simulink model "diabetes_2sim"  (R2019a)
settings: Solver=ode45  StartTime=0.0  StopTime=24  RelTol=1e-3  EnableMultiTasking=on
StopFcn:
  | plot_results
libraries: simulink x2, realtime_pacer_lib x1
settings Model: Creator=tsladeche  LastModifiedBy=esthe
settings DataIOCC: LimitDataPoints=on  SaveFormat=Array  SignalLoggingSaveFormat=ModelDataLogs  ReturnWorkspaceOutputs=off
settings OptimizationCC: ExpressionDepthLimit=2147483647  LifeSpan=inf
settings DebuggingCC: UnderspecifiedInitializationDetection=Classic  MergeDetectMultiDrivingBlocksExec=none  SolverPrmCheckMsg=warning  FcnCallInpInsideContextMsg=warning  StateNameClashWarn=warning  SFUnexpectedBacktrackingDiag=warning  SFNoUnconditionalDefaultTransitionDiag=warning  SFExecutionAtInitializationDiag=none  ArithmeticOperatorsInVariantConditions=warning
settings HardwareCC: ProdBitPerPointer=32  ProdBitPerSizeT=32  ProdBitPerPtrDiffT=32  ProdLargestAtomicFloat=None  ProdIntDivRoundTo=Undefined  ProdEndianess=Unspecified  ProdWordSize=32  ProdHWDeviceType=32-bit Generic
settings ModelReferenceCC: PropagateSignalLabelsOutOfModel=off
settings SFSimCC: SimUseLocalCustomCode=off
settings RTWCC: RTWUseLocalCustomCode=off
settings CodeAppCC: StateflowObjectComments=on
settings GRTTargetCC: TargetLangStandard=C89/C90 (ANSI)  GeneratePreprocessorConditionals=Disable all  CombineOutputUpdateFcns=off  GRTInterface=on
settings ConfigComp: CovMetricSettings=dw  CovHtmlReporting=on  CovSaveCumulativeToWorkspaceVar=on  CovSaveSingleToWorkspaceVar=on  CovExternalEMLEnable=off

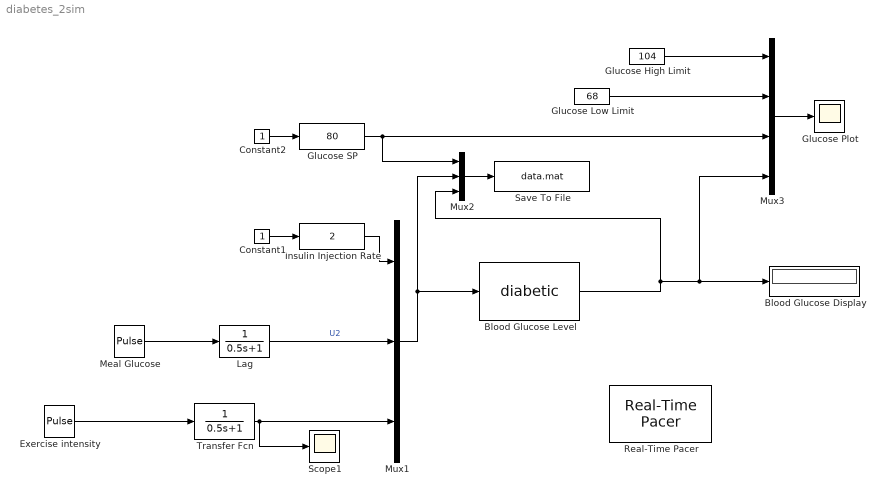
== system diabetes_2sim ==
  Blood Glucose Display : Display
  Blood Glucose Level : S-Function  FunctionName=diabetic  SFunctionDeploymentMode=off  EnableBusSupport=off
  Constant1 : Constant
  Constant2 : Constant
  Exercise intensity : DiscretePulseGenerator  PulseType=Time based  Amplitude=40  Period=24  PulseWidth=10  PhaseDelay=4
  Glucose High Limit : Constant  Value=104
  Glucose Low Limit : Constant  Value=68
  Glucose Plot : Scope
  Glucose SP : simulink/Math Operations/Slider Gain  gain=80  low=50  high=120
  Insulin Injection Rate : simulink/Math Operations/Slider Gain  gain=2  low=0  high=10
  Lag : TransferFcn  Denominator=[0.5 1]
  Meal Glucose : DiscretePulseGenerator  PulseType=Time based  Amplitude=50  Period=6  PulseWidth=10  PhaseDelay=8
  Mux1 : Mux  Inputs=3
  Mux2 : Mux  Inputs=3
  Mux3 : Mux
  Real-Time Pacer : realtime_pacer_lib/Real-Time Pacer  simTimePerRealTime=1.0
  Save To File : ToFile  Filename=data.mat  MatrixName=diabetic  SampleTime=0.05
  Scope1 : Scope
  Transfer Fcn : TransferFcn  Denominator=[0.5 1]
  wires:
  Mux2/1 -> Save To File/1
  Constant1/1 -> Insulin Injection Rate/1
  Mux1/1 -> Blood Glucose Level/1, Mux2/2
  Constant2/1 -> Glucose SP/1
  Glucose SP/1 -> Mux3/3, Mux2/1
  Blood Glucose Level/1 -> Mux3/4, Blood Glucose Display/1, Mux2/3
  Glucose High Limit/1 -> Mux3/1
  Glucose Low Limit/1 -> Mux3/2
  Mux3/1 -> Glucose Plot/1
  Insulin Injection Rate/1 -> Mux1/1
  Meal Glucose/1 -> Lag/1
  Lag/1 -> Mux1/2  "U2"
  Exercise intensity/1 -> Transfer Fcn/1
  Transfer Fcn/1 -> Scope1/1, Mux1/3
